simulink model "inverted_pend_2"  (R2020a)
settings: Solver=VariableStepAuto  StartTime=0.0  StopTime=15  RelTol=1e-3
values from neighbouring files (symbols this model uses):
  D = 0    [compute_cart_pole_linear_system.m]    (also in rscale.m = d)
  g = p.g    [compute_cart_pole_linear_system.m]    (also in set_parameters.m; test_mpc.m = 9.81)
  I_rotor = p.I_rotor    [compute_cart_pole_linear_system.m]    (also in set_parameters.m; test_mpc.m = 7e-06)
  Kt = p.Kt    [compute_cart_pole_linear_system.m]    (also in set_parameters.m; test_mpc.m = 0.0135)
  Kv = p.Kv    [compute_cart_pole_linear_system.m]    (also in set_parameters.m; test_mpc.m = 0.0186)
  l = 0.3    [animate_system.m]    (also in compute_cart_pole_linear_system.m = p.l; set_parameters.m = p.l; test_mpc.m)
  M = p.M    [compute_cart_pole_linear_system.m]    (also in set_parameters.m; test_mpc.m = 0.5)
  m = p.m    [compute_cart_pole_linear_system.m]    (also in set_parameters.m; test_mpc.m = 0.2)
  N_rotor = p.N_rotor    [compute_cart_pole_linear_system.m]    (also in set_parameters.m; test_mpc.m = 26.9)
  r_pulley = p.r_pulley    [compute_cart_pole_linear_system.m]    (also in set_parameters.m; test_mpc.m = 0.006)
  Rw = p.Rw    [compute_cart_pole_linear_system.m]    (also in set_parameters.m; test_mpc.m = 1.3)
  x_desired = 0.5    [MAIN.m]
libraries: mpclib x1, cstblocks x1
settings Model: Creator=Leo Song  LastModifiedBy=Leo Song

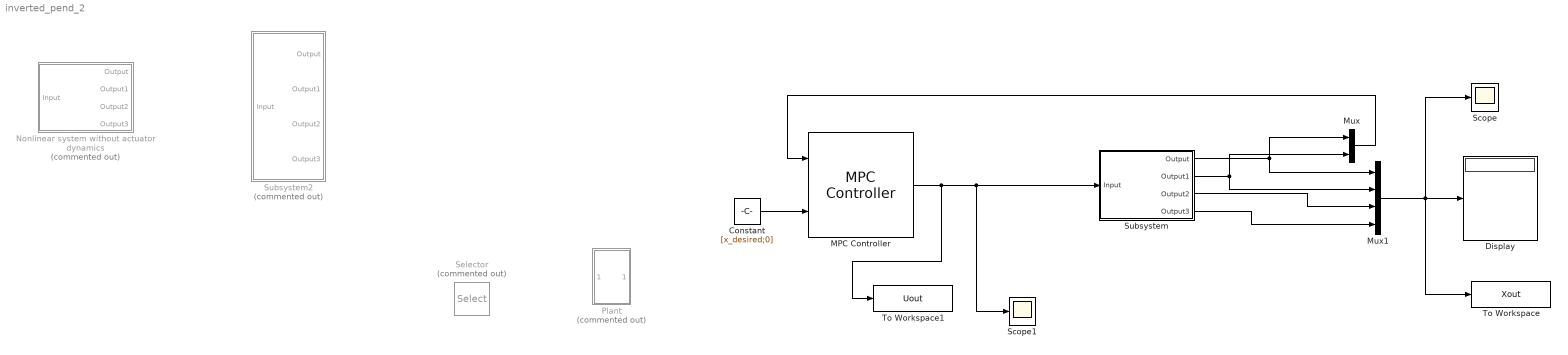
== system inverted_pend_2 ==
  Constant : Constant  Value=[x_desired;0]
  Display : Display
  MPC Controller : mpclib/MPC Controller  SCDEnableBlockLinearizationSpecification=on  mpcobj=mpc1  is_multiple=0  enable_value=0  return_u0=off  updateMPCinCallerWorkspace=on  md_inport=off  mv_inport=off  uref_inport=off  return_cost=off  return_mvseq=off  return_qpstatus=off  return_xseq=off  return_state=off  return_ovseq=off  state_inport=off  umin_inport=off  umax_inport=off  ymin_inport=off  ymax_inport=off  cc_inport=off  ywt_inport=off  uwt_inport=off  duwt_inport=off  rhoeps_inport=off  pm_inport=off  MaximumP=10  HorizonChoice=FixedHorizon  n_ts=0.001  n_p=4000  n_mv=1  n_md=0  n_ud=0  n_mo=2  n_uo=0  BlockDataType=double  SampleTimeInherited=off  switch_inport=off
  Mux : Mux  Inputs=2
  Mux1 : Mux
  Nonlinear system without actuator dynamics : Subsystem  Commented=on
  Plant : Subsystem  Commented=on
  Scope : Scope
  Scope1 : Scope
  Selector : Selector  Commented=on  InputPortWidth=4  IndexOptions=Index vector (dialog)  Indices=[1 2]  OutputSizes=1
  Subsystem : Subsystem
  Subsystem2 : Subsystem  Commented=on
  To Workspace : ToWorkspace  VariableName=Xout  SampleTime=-1
  To Workspace1 : ToWorkspace  VariableName=Uout  SampleTime=-1
  wires:
  Constant/1 -> MPC Controller/2
  MPC Controller/1 -> To Workspace1/1, Scope1/1, Subsystem/1(Input)
  Mux/1 -> MPC Controller/1
  Mux1/1 -> To Workspace/1, Scope/1, Display/1
  Subsystem/1(Output) -> Mux1/1, Mux/1
  Subsystem/2(Output1) -> Mux1/2, Mux/2
  Subsystem/3(Output2) -> Mux1/3
  Subsystem/4(Output3) -> Mux1/4

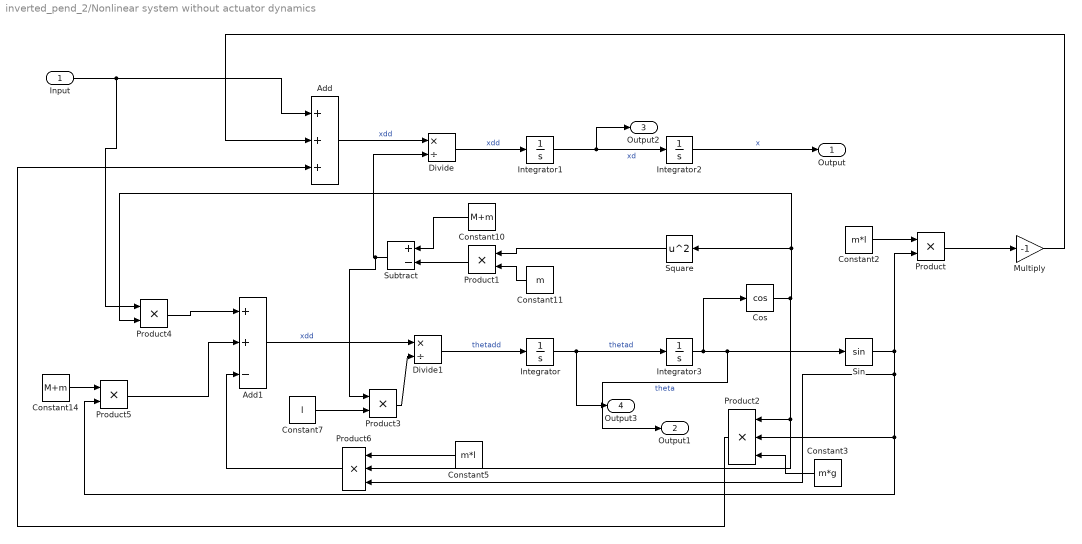
== system inverted_pend_2/Nonlinear system without actuator dynamics ==
  Input : Inport
  Add : Sum  Inputs=+++
  Add1 : Sum  Inputs=++-
  Constant10 : Constant  Value=M+m
  Constant11 : Constant  Value=m
  Constant14 : Constant  Value=M+m
  Constant2 : Constant  Value=m*l
  Constant3 : Constant  Value=m*g
  Constant5 : Constant  Value=m*l
  Constant7 : Constant  Value=l
  Cos : Trigonometry  Operator=cos
  Divide : Product  Inputs=*/
  Divide1 : Product  Inputs=*/
  Integrator{,1..3} (4 alike) : Integrator
  Multiply : Gain  Gain=-1
  Product{,1,3..5} (5 alike) : Product
  Product2 : Product  Inputs=3
  Product6 : Product  Inputs=3
  Sin : Trigonometry
  Square : Math  Operator=square  SaturateOnIntegerOverflow=on
  Subtract : Sum  Inputs=+-
  Output : Outport
  Output1 : Outport  Port=2
  Output2 : Outport  Port=3
  Output3 : Outport  Port=4
  wires:
  Constant14/1 -> Product5/1
  Constant5/1 -> Product6/1
  Divide1/1 -> Integrator/1  "thetadd"
  Constant7/1 -> Product3/2
  Subtract/1 -> Product3/1, Divide/2
  Integrator2/1 -> Output/1  "x"
  Integrator/1 -> Output3/1, Integrator3/1  "thetad"
  Add/1 -> Divide/1  "xdd"
  Divide/1 -> Integrator1/1  "xdd"
  Integrator1/1 -> Output2/1, Integrator2/1  "xd"
  Input/1 -> Product4/1, Add/1
  Sin/1 -> Product6/3, Product5/2, Product2/2, Product/2
  Product6/1 -> Add1/3
  Cos/1 -> Product6/2, Product2/1, Product4/2, Square/1
  Integrator3/1 -> Cos/1, Output1/1, Sin/1  "theta"
  Constant3/1 -> Product2/3
  Constant2/1 -> Product/1
  Product/1 -> Multiply/1
  Product3/1 -> Divide1/2
  Product5/1 -> Add1/2
  Constant10/1 -> Subtract/1
  Product1/1 -> Subtract/2
  Square/1 -> Product1/1
  Constant11/1 -> Product1/2
  Product2/1 -> Add/3
  Add1/1 -> Divide1/1  "xdd"
  Product4/1 -> Add1/1
  Multiply/1 -> Add/2

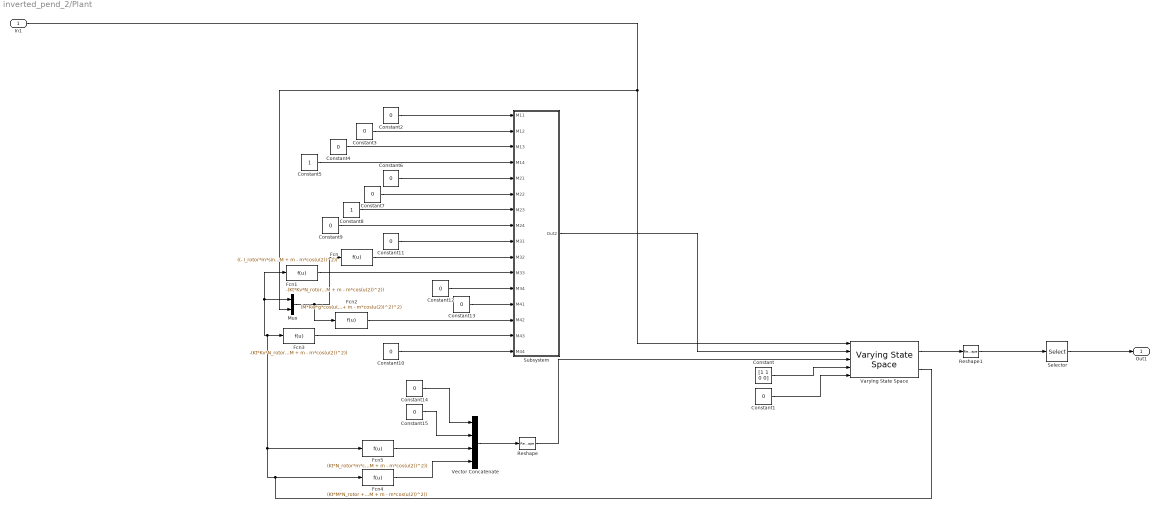
== system inverted_pend_2/Plant ==
  In1 : Inport
  Constant : Constant  Value=[1 1 0 0]
  Constant{1..4,6..7,9..15} (13 alike) : Constant  Value=0
  Constant5 : Constant
  Constant8 : Constant
  Fcn : Fcn  Expr=((- I_rotor*m*sin(u(2))*N_rotor^2*r_pulley^2 + 2*m*cos(u(2))*sin(u(2)))*(Kt*Kv*m*u(3)*cos(u(2))*N_rotor^2 - Kt*m*u(5)*cos(u(2))*N_rotor + Rw*l*m*sin(u(2)) - Rw*g*m*cos(u(2))*sin(u(2))))/(Rw*(I_rotor*m*cos(u(2))*N_rotor^2*r_pulley^2 + M + m - m*cos(u(2))^2)^2) - (Rw*l*m*cos(u(2)) - Rw*g*m*cos(u(2))^2 + Rw*g*m*sin(u(2))^2 + Kt*N_rotor*m*u(5)*sin(u(2)) - Kt*Kv*N_rotor^2*m*u(3)*sin(u(2)))/(Rw*(I_rotor*m*cos(u(2))*N_rotor^2*r_pulley^2 + M + m - m*cos(u(2))^2))
  Fcn1 : Fcn  Expr=-(Kt*Kv*N_rotor^2*m*cos(u(2)))/(Rw*(I_rotor*m*cos(u(2))*N_rotor^2*r_pulley^2 + M + m - m*cos(u(2))^2))
  Fcn2 : Fcn  Expr=(M*Rw*g*cos(u(2)) + Rw*g*m*cos(u(2)) - Rw*l*m*cos(u(2))^2 + Rw*l*m*sin(u(2))^2 + I_rotor*N_rotor^2*Rw*l*m*r_pulley^2*cos(u(2)))/(Rw*l*(I_rotor*m*cos(u(2))*N_rotor^2*r_pulley^2 + M + m - m*cos(u(2))^2)) - ((- I_rotor*m*sin(u(2))*N_rotor^2*r_pulley^2 + 2*m*cos(u(2))*sin(u(2)))*(M*Rw*g*sin(u(2)) + Rw*g*m*sin(u(2)) + Kt*M*N_rotor*u(5) + Kt*N_rotor*m* u(5) - Rw*l*m*cos(u(2))*sin(u(2)) - Kt*Kv*M*N_rotor^2*u(3) - Kt*Kv*N_rotor^2*m*u(3) + I_rotor*N_rotor^2*Rw*l*m*r_pulley^2*sin(u(2))))/(Rw*l*(I_rotor*m*cos(u(2))*N_rotor^2*r_pulley^2 + M + m - m*cos(u(2))^2)^2)
  Fcn3 : Fcn  Expr=-(Kt*Kv*N_rotor^2*m + Kt*Kv*M*N_rotor^2)/(Rw*l*(I_rotor*m*cos(u(2))*N_rotor^2*r_pulley^2 + M + m - m*cos(u(2))^2))
  Fcn4 : Fcn  Expr=(Kt*M*N_rotor + Kt*N_rotor*m)/(Rw*l*(I_rotor*m*cos(u(2))*N_rotor^2*r_pulley^2 + M + m - m*cos(u(2))^2))
  Fcn5 : Fcn  Expr=(Kt*N_rotor*m*cos(u(2)))/(Rw*(I_rotor*m*cos(u(2))*N_rotor^2*r_pulley^2 + M + m - m*cos(u(2))^2))
  Mux : Mux  Inputs=2
  Reshape : Reshape  OutputDimensionality=Column vector (2-D)  OutputDimensions=[4,1]
  Reshape1 : Reshape  OutputDimensionality=Column vector (2-D)
  Selector : Selector  InputPortWidth=16  IndexOptions=Index vector (dialog)  Indices=[1 5 9 13]  OutputSizes=1
  Subsystem : Subsystem
  Varying State Space : cstblocks/Linear Parameter Varying/Varying State Space  x0=[0, 0.0, 0.00, 0.0]  xNames=['x','theta','x_dot','theta_dot']  OutputX=on  OutputDX=off
  Vector Concatenate : Concatenate  NumInputs=4
  Out1 : Outport
  wires:
  Fcn3/1 -> Subsystem/15(M43)
  Mux/1 -> Fcn/1, Fcn2/1
  Constant12/1 -> Subsystem/12(M34)
  Constant13/1 -> Subsystem/13(M41)
  Constant2/1 -> Subsystem/1(M11)
  Fcn2/1 -> Subsystem/14(M42)
  Constant9/1 -> Subsystem/8(M24)
  Constant3/1 -> Subsystem/2(M12)
  In1/1 -> Mux/2, Varying State Space/1
  Varying State Space/2 -> Fcn5/1, Mux/1, Fcn1/1, Fcn3/1, Fcn4/1
  Constant/1 -> Varying State Space/4
  Subsystem/1(Out2) -> Varying State Space/2
  Constant8/1 -> Subsystem/7(M23)
  Fcn/1 -> Subsystem/10(M32)
  Constant11/1 -> Subsystem/9(M31)
  Constant7/1 -> Subsystem/6(M22)
  Fcn5/1 -> Vector Concatenate/3
  Constant5/1 -> Subsystem/4(M14)
  Fcn1/1 -> Subsystem/11(M33)
  Reshape1/1 -> Selector/1
  Constant4/1 -> Subsystem/3(M13)
  Constant6/1 -> Subsystem/5(M21)
  Constant14/1 -> Vector Concatenate/1
  Constant15/1 -> Vector Concatenate/2
  Constant1/1 -> Varying State Space/5
  Fcn4/1 -> Vector Concatenate/4
  Selector/1 -> Out1/1
  Varying State Space/1 -> Reshape1/1
  Reshape/1 -> Varying State Space/3
  Constant10/1 -> Subsystem/16(M44)
  Vector Concatenate/1 -> Reshape/1

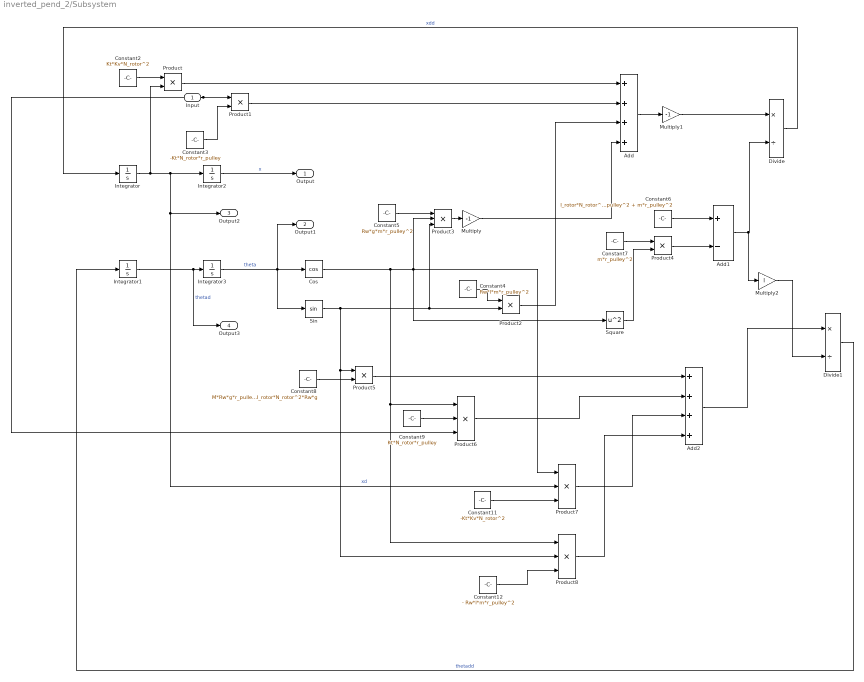
== system inverted_pend_2/Subsystem ==
  Input : Inport
  Add : Sum  Inputs=++++
  Add1 : Sum  Inputs=+-
  Add2 : Sum  Inputs=++++
  Constant11 : Constant  Value=-Kt*Kv*N_rotor^2
  Constant12 : Constant  Value=- Rw*l*m*r_pulley^2
  Constant2 : Constant  Value=Kt*Kv*N_rotor^2
  Constant3 : Constant  Value=-Kt*N_rotor*r_pulley
  Constant4 : Constant  Value=Rw*l*m*r_pulley^2
  Constant5 : Constant  Value=Rw*g*m*r_pulley^2
  Constant6 : Constant  Value=I_rotor*N_rotor^2 + M*r_pulley^2 + m*r_pulley^2
  Constant7 : Constant  Value=m*r_pulley^2
  Constant8 : Constant  Value=M*Rw*g*r_pulley^2+Rw*g*m*r_pulley^2+I_rotor*N_rotor^2*Rw*g
  Constant9 : Constant  Value=Kt*N_rotor*r_pulley
  Cos : Trigonometry  Operator=cos
  Divide : Product  Inputs=*/
  Divide1 : Product  Inputs=*/
  Integrator{,1..3} (4 alike) : Integrator
  Multiply : Gain  Gain=-1
  Multiply1 : Gain  Gain=-1
  Multiply2 : Gain  Gain=l
  Product{,1..2,4..5} (5 alike) : Product
  Product{3,6..8} (4 alike) : Product  Inputs=3
  Sin : Trigonometry
  Square : Math  Operator=square  SaturateOnIntegerOverflow=on
  Output : Outport
  Output1 : Outport  Port=2
  Output2 : Outport  Port=3
  Output3 : Outport  Port=4
  wires:
  Product4/1 -> Add1/2
  Product8/1 -> Add2/4
  Divide/1 -> Integrator/1  "xdd"
  Sin/1 -> Product8/2, Product5/1, Product3/3, Product2/2
  Integrator/1 -> Product/2, Output2/1, Product7/2, Integrator2/1  "xd"
  Constant5/1 -> Product3/1
  Constant4/1 -> Product2/1
  Constant8/1 -> Product5/2
  Integrator3/1 -> Output1/1, Sin/1, Cos/1  "theta"
  Product6/1 -> Add2/2
  Cos/1 -> Product8/1, Product6/1, Product7/1, Product3/2, Square/1
  Constant3/1 -> Product1/2
  Constant11/1 -> Product7/3
  Integrator2/1 -> Output/1  "x"
  Multiply/1 -> Add/4
  Constant9/1 -> Product6/2
  Constant6/1 -> Add1/1
  Product3/1 -> Multiply/1
  Product1/1 -> Add/2
  Constant12/1 -> Product8/3
  Add1/1 -> Multiply2/1, Divide/2
  Add2/1 -> Divide1/1
  Constant2/1 -> Product/1
  Product7/1 -> Add2/3
  Input/1 -> Product1/1, Product6/3
  Constant7/1 -> Product4/1
  Square/1 -> Product4/2
  Product2/1 -> Add/3
  Integrator1/1 -> Output3/1, Integrator3/1  "thetad"
  Divide1/1 -> Integrator1/1  "thetadd"
  Multiply2/1 -> Divide1/2
  Product5/1 -> Add2/1
  Multiply1/1 -> Divide/1
  Product/1 -> Add/1
  Add/1 -> Multiply1/1

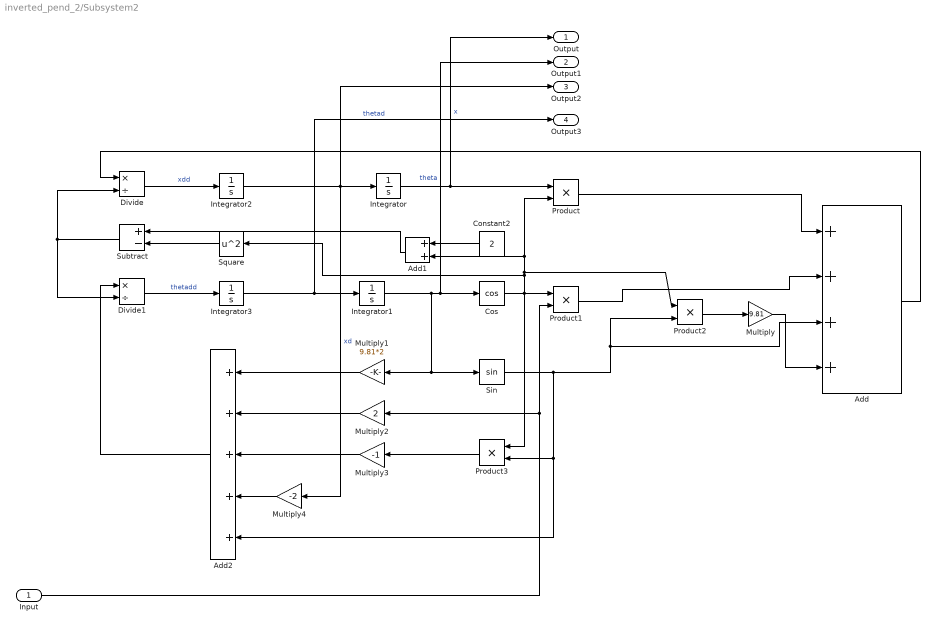
== system inverted_pend_2/Subsystem2 ==
  Input : Inport
  Add : Sum  Inputs=++++
  Add1 : Sum
  Add2 : Sum  Inputs=+++++
  Constant2 : Constant  Value=2
  Cos : Trigonometry  Operator=cos
  Divide : Product  Inputs=*/
  Divide1 : Product  Inputs=*/
  Integrator{,1..3} (4 alike) : Integrator
  Multiply : Gain  Gain=9.81
  Multiply1 : Gain  Gain=9.81*2
  Multiply2 : Gain  Gain=2
  Multiply3 : Gain  Gain=-1
  Multiply4 : Gain  Gain=-2
  Product{,1..3} (4 alike) : Product
  Sin : Trigonometry
  Square : Math  Operator=square  SaturateOnIntegerOverflow=on
  Subtract : Sum  Inputs=+-
  Output : Outport
  Output1 : Outport  Port=2
  Output2 : Outport  Port=3
  Output3 : Outport  Port=4
  wires:
  Multiply1/1 -> Add2/1
  Sin/1 -> Add2/5, Product3/2, Product2/2, Add/3
  Integrator2/1 -> Output2/1, Multiply4/1, Integrator/1  "xd"
  Subtract/1 -> Divide1/2, Divide/2
  Multiply2/1 -> Add2/2
  Integrator3/1 -> Output3/1, Integrator1/1  "thetad"
  Multiply/1 -> Add/4
  Add2/1 -> Divide1/1
  Integrator/1 -> Output/1, Product/1  "x"
  Square/1 -> Subtract/2
  Cos/1 -> Product3/1, Product1/1, Square/1, Product2/1, Add1/2, Product/2
  Constant2/1 -> Add1/1
  Input/1 -> Product1/2, Multiply2/1
  Add/1 -> Divide/1
  Product/1 -> Add/1
  Product1/1 -> Add/2
  Divide1/1 -> Integrator3/1  "thetadd"
  Multiply4/1 -> Add2/4
  Integrator1/1 -> Output1/1, Cos/1, Multiply1/1, Sin/1  "theta"
  Multiply3/1 -> Add2/3
  Divide/1 -> Integrator2/1  "xdd"
  Product3/1 -> Multiply3/1
  Add1/1 -> Subtract/1
  Product2/1 -> Multiply/1

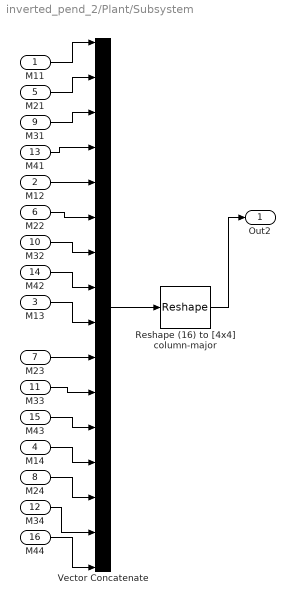
== system inverted_pend_2/Plant/Subsystem ==
  M11 : Inport  PortDimensions=1
  M12 : Inport  Port=2  PortDimensions=1
  M13 : Inport  Port=3  PortDimensions=1
  M14 : Inport  Port=4  PortDimensions=1
  M21 : Inport  Port=5  PortDimensions=1
  M22 : Inport  Port=6  PortDimensions=1
  M23 : Inport  Port=7  PortDimensions=1
  M24 : Inport  Port=8  PortDimensions=1
  M31 : Inport  Port=9  PortDimensions=1
  M32 : Inport  Port=10  PortDimensions=1
  M33 : Inport  Port=11  PortDimensions=1
  M34 : Inport  Port=12  PortDimensions=1
  M41 : Inport  Port=13  PortDimensions=1
  M42 : Inport  Port=14  PortDimensions=1
  M43 : Inport  Port=15  PortDimensions=1
  M44 : Inport  Port=16  PortDimensions=1
  Reshape (16) to [4x4] column-major : Reshape  OutputDimensionality=Customize  OutputDimensions=[4,4]
  Vector Concatenate : Concatenate  NumInputs=16
  Out2 : Outport
  wires:
  M14/1 -> Vector Concatenate/13
  M13/1 -> Vector Concatenate/9
  M33/1 -> Vector Concatenate/11
  M21/1 -> Vector Concatenate/2
  M22/1 -> Vector Concatenate/6
  M43/1 -> Vector Concatenate/12
  M23/1 -> Vector Concatenate/10
  Reshape (16) to [4x4] column-major/1 -> Out2/1
  Vector Concatenate/1 -> Reshape (16) to [4x4] column-major/1
  M11/1 -> Vector Concatenate/1
  M42/1 -> Vector Concatenate/8
  M34/1 -> Vector Concatenate/15
  M44/1 -> Vector Concatenate/16
  M12/1 -> Vector Concatenate/5
  M32/1 -> Vector Concatenate/7
  M41/1 -> Vector Concatenate/4
  M24/1 -> Vector Concatenate/14
  M31/1 -> Vector Concatenate/3
